simulink model "closed_loop_withSA60"  (R2015a)
settings: Solver=ode45  StartTime=0.0  StopTime=.25  RelTol=1e-9
settings Model: ExtModeAutoUpdateStatusClock=off  Creator=wrmurray  LastModifiedBy=melab15
settings DataIOCC: LimitDataPoints=off  SignalLoggingSaveFormat=ModelDataLogs  Refine=2
settings OptimizationCC: ExpressionDepthLimit=2147483647  InitFltsAndDblsToZero=on
settings DebuggingCC: SaveWithParameterizedLinksMsg=none  UnderspecifiedInitializationDetection=Classic  MergeDetectMultiDrivingBlocksExec=none  SignalResolutionControl=TryResolveAllWithWarning  SolverPrmCheckMsg=warning  MultiTaskDSMMsg=warning  MultiTaskCondExecSysMsg=none  FcnCallInpInsideContextMsg=UseLocalSettings  StateNameClashWarn=warning
settings GRTTargetCC: TargetFcnLib=ansi_tfl_tmw.mat  CombineOutputUpdateFcns=off  GRTInterface=on

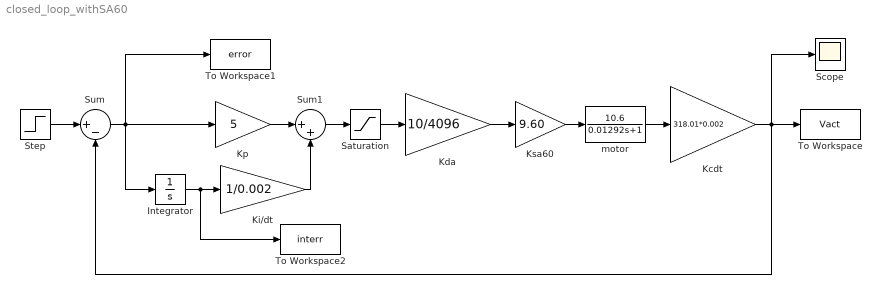
== system closed_loop_withSA60 ==
  Integrator : Integrator
  Kcdt : Gain  Gain=318.01*0.002
  Kda : Gain  Gain=10/4096
  Ki/dt : Gain  Gain=1/0.002
  Kp : Gain  Gain=5
  Ksa60 : Gain  Gain=9.60
  Saturation : Saturate  UpperLimit=1024  LowerLimit=-1024
  Scope : Scope
      settings: TimeRange=0.1
  Step : Step  Time=.014  After=100  SampleTime=0
  Sum : Sum  Inputs=|+-
  Sum1 : Sum  Inputs=|++
  To Workspace : ToWorkspace  VariableName=Vact  SampleTime=-1
  To Workspace1 : ToWorkspace  VariableName=error  SampleTime=-1
  To Workspace2 : ToWorkspace  VariableName=interr  SampleTime=-1
  motor : TransferFcn  Numerator=[10.6]  Denominator=[0.01292 1]
  wires:
  Sum/1 -> Kp/1, To Workspace1/1, Integrator/1
  Ksa60/1 -> motor/1
  motor/1 -> Kcdt/1
  Kcdt/1 -> Sum/2, Scope/1, To Workspace/1
  Saturation/1 -> Kda/1
  Kda/1 -> Ksa60/1
  Integrator/1 -> Ki/dt/1, To Workspace2/1
  Kp/1 -> Sum1/1
  Sum1/1 -> Saturation/1
  Ki/dt/1 -> Sum1/2
  Step/1 -> Sum/1
